simulink model "drone"  (R2019a)
settings: Solver=VariableStepAuto  StartTime=0.0  StopTime=50.0  RelTol=1e-3
settings Model: Creator=hansae  LastModifiedBy=hansae
settings DebuggingCC: UnconnectedInputMsg=none  UnconnectedOutputMsg=none  UnconnectedLineMsg=none  SFMachineParentedDataDiag=error
settings ModelReferenceCC: EnableRefExpFcnMdlSchedulingChecks=off
settings RTWCC: Description=Generic Real-Time Target

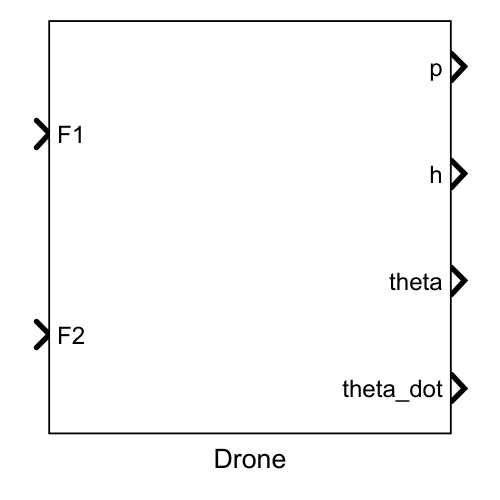
[thumbnail: Simulink's stored preview of the top-level diagram]
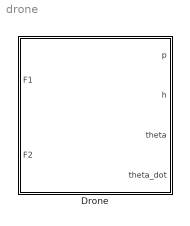
== system drone ==
  Drone : Subsystem

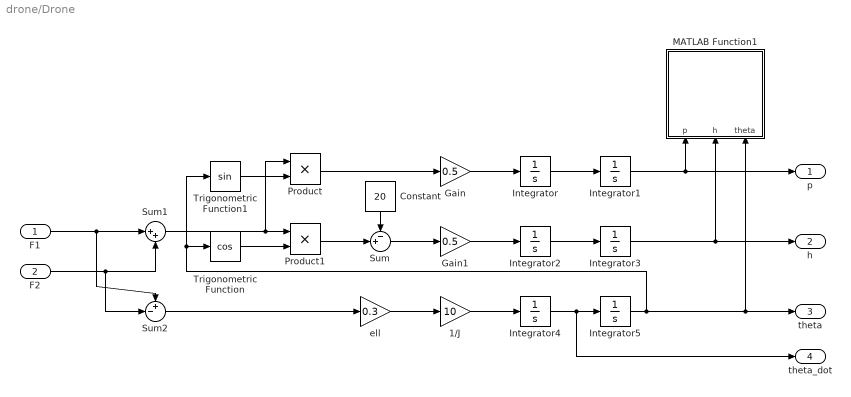
== system drone/Drone ==
  F1 : Inport
  F2 : Inport  Port=2
  1/J : Gain  Gain=10
  Constant : Constant  Value=20
  Gain : Gain  Gain=0.5
  Gain1 : Gain  Gain=0.5
  Integrator{,1..2,4..5} (5 alike) : Integrator
  Integrator3 : Integrator  LimitOutput=on  LowerSaturationLimit=0
  MATLAB Function1 : MATLAB Function  TreatAsAtomicUnit=on  SystemSampleTime=1/30
  Product : Product
  Product1 : Product
  Sum : Sum  Inputs=-+|
  Sum1 : Sum  Inputs=|++
  Sum2 : Sum  Inputs=+-|
  Trigonometric Function : Trigonometry  Operator=cos
  Trigonometric Function1 : Trigonometry
  ell : Gain  Gain=0.3
  p : Outport
  h : Outport  Port=2
  theta : Outport  Port=3
  theta_dot : Outport  Port=4
  wires:
  Integrator3/1 -> h/1, MATLAB Function1/2(h)
  Integrator5/1 -> MATLAB Function1/3(theta), theta/1, Trigonometric Function/1, Trigonometric Function1/1
  Trigonometric Function/1 -> Product1/2
  Integrator4/1 -> theta_dot/1, Integrator5/1
  Product/1 -> Gain/1
  Integrator1/1 -> MATLAB Function1/1(p), p/1
  Sum2/1 -> ell/1
  1/J/1 -> Integrator4/1
  Sum/1 -> Gain1/1
  Trigonometric Function1/1 -> Product/2
  Integrator2/1 -> Integrator3/1
  Integrator/1 -> Integrator1/1
  Gain/1 -> Integrator/1
  F2/1 -> Sum2/2, Sum1/2
  Gain1/1 -> Integrator2/1
  F1/1 -> Sum2/1, Sum1/1
  Sum1/1 -> Product/1, Product1/1
  ell/1 -> 1/J/1
  Constant/1 -> Sum/1
  Product1/1 -> Sum/2

== matlab function drone/Drone/MATLAB Function1 ==
  settings: updateMethod=DISCRETE
  data: p input; h input; theta input
function plot_drone(p, h, theta)
    % Constants
    N = 40;
    ell = 0.3;

    % Persistent variables
    persistent buffer_p buffer_h writeIdx iter;
    persistent Drone Trace_vector;
    
    % Initialize iteration count
    if isempty(iter)
        iter = 0;
    else
        iter = iter + 1;
    end

    % Buffer Initialization
    if isempty(buffer_p)
        buffer_p = zeros(N, 1);
        buffer_h = zeros(N, 1);
        writeIdx = 1;
    elseif mod(iter, 2) == 0
        buffer_p(writeIdx) = p;
        buffer_h(writeIdx) = h;
        writeIdx = mod(writeIdx, N) + 1;
    end

    % Drone Plot Initialization
    if isempty(Drone)
        Drone = initialize_plot(ell);
    else
        update_drone_position(Drone, p, h, theta);
        drawnow;
    end

    % Trace Vector Initialization
    if isempty(Trace_vector)
        Trace_vector = [hgtransform('parent', gca)];
        for i = 1:N
            Trace_vector = [Trace_vector, hgtransform('parent', gca)];
            plot(0, 0, 'r.', 'markersize', 10, 'Parent', Trace_vector(i));
        end
    elseif mod(iter, 2) == 0
        for i = 1:N
            if ishandle(Trace_vector(i))
                set(Trace_vector(i), 'Matrix', makehgtform('translate', [buffer_p(i), buffer_h(i), 0]));
            end
        end
    end
    
    %% Nested functions
    function Drone = initialize_plot(ell)
        % Setup figure
        figure(1); clf; grid on; hold on; daspect([1, 1, 1]);
        xlim([-2*ell, 2*ell]);
        ylim([-2*ell, 2*ell]);
        xlabel('$p$','interpreter','latex')
        ylabel('$h$','interpreter','latex')

        
        % Draw ground
        yline(-0.47*ell, 'k', 'linewidth', 3);
        
        % Draw drones
        Drone = draw_drone(p, h, ell, 1);
    end

    function update_drone_position(Drone, p, h, theta)
        if ishandle(Drone)
            set(Drone, 'Matrix', makehgtform('translate', [p, h, 0], 'zrotate', -theta));
            xlim([-2*ell, 2*ell] + p);
            ylim([-2*ell, 2*ell] + h);
        end
    end

    function Drone = draw_drone(p,h,ell,opacity)
        % Derived parameters
        w_body = 2*0.27*ell;
        h_body = w_body/2;
        w_prop_body = h_body/2;
        h_prop_body = w_prop_body;
        h_prop_triangle = h_prop_body;
        r_prop = w_body/2;
        dp_feet = 0.4*ell;
        dh_feet = 0.47*ell;
        r_feet = 0.01*ell/0.3;
        r_center = 0.015*ell/0.3;    
        linewidth_narrow = 1;
        linewidth_wide = 2;

        % Drone
        Drone = hgtransform('parent',gca);
        
        % Props
        rectangle('Position',[p+ell-w_prop_body/2,h-h_prop_body,w_prop_body,h_prop_body],'Edgecolor', [0,0,0,opacity],'FaceColor',[1,1,1,opacity],'linewidth',linewidth_narrow,'Parent',Drone);
        rectangle('Position',[p-ell-w_prop_body/2,h-h_prop_body,w_prop_body,h_prop_body],'Edgecolor', [0,0,0,opacity],'FaceColor',[1,1,1,opacity],'linewidth',linewidth_narrow,'Parent',Drone);
        fill([p+ell+w_prop_body/2, p+ell, p+ell-w_prop_body/2, p+ell+w_prop_body/2], [h, h+h_prop_triangle, h, h],'w','FaceAlpha',opacity,'EdgeAlpha',opacity,'linewidth',linewidth_narrow,'Parent',Drone);
        fill([p-ell+w_prop_body/2, p-ell, p-ell-w_prop_body/2, p-ell+w_prop_body/2], [h, h+h_prop_triangle, h, h],'w','FaceAlpha',opacity,'EdgeAlpha',opacity,'linewidth',linewidth_narrow,'Parent',Drone);
        line([p+ell-r_prop, p+ell+r_prop], [h+2*h_prop_triangle/4, h+2*h_prop_triangle/4],'linewidth',linewidth_narrow,'color',[0,0,0,opacity],'Parent',Drone);
        line([p-ell-r_prop, p-ell+r_prop], [h+2*h_prop_triangle/4, h+2*h_prop_triangle/4],'linewidth',linewidth_narrow,'color',[0,0,0,opacity],'Parent',Drone);
        
        % Feet
        alpha = 0.28; % Hack to fix feet being visible through body when transparent
        line([p+alpha*dp_feet,p+dp_feet],[h-alpha*dh_feet,h-dh_feet],'linewidth',linewidth_narrow,'color',[0,0,0,opacity],'Parent',Drone);
        line([p-alpha*dp_feet,p-dp_feet],[h-alpha*dh_feet,h-dh_feet],'linewidth',linewidth_narrow,'color',[0,0,0,opacity],'Parent',Drone);
        rectangle('Position',[p+dp_feet-r_feet/2,h-dh_feet-r_feet/2,r_feet,r_feet],'Curvature',1,'Edgecolor', [0,0,0,opacity],'FaceColor',[0,0,0,opacity],'linewidth',linewidth_narrow,'Parent',Drone);
        rectangle('Position',[p-dp_feet-r_feet/2,h-dh_feet-r_feet/2,r_feet,r_feet],'Curvature',1,'Edgecolor', [0,0,0,opacity],'FaceColor',[0,0,0,opacity],'linewidth',linewidth_narrow,'Parent',Drone);
        
        % Arms
        line([p+w_body/2,p+ell+w_prop_body/2],[0,0],'linewidth',linewidth_wide,'color',[0,0,0,opacity],'Parent',Drone);
        line([p-w_body/2,p-ell-w_prop_body/2],[0,0],'linewidth',linewidth_wide,'color',[0,0,0,opacity],'Parent',Drone);
        
        % Body
        rectangle('Position',[p-w_body/2,h-h_body/2,w_body,h_body],'Edgecolor', [0,0,0,opacity],'FaceColor',[1,1,1,opacity],'linewidth',linewidth_narrow,'Parent',Drone);
        rectangle('Position',[p-r_center/2,h-r_center/2,r_center,r_center],'Curvature',1,'Edgecolor', [0,0,0,opacity],'FaceColor',[0,0,0,opacity],'linewidth',linewidth_narrow,'Parent',Drone);
    end
end
